simulink model "Task_Stable"  (R2023a)
settings: Solver=VariableStepAuto  StartTime=0.0  StopTime=10.0  RelTol=1e-3
libraries: cstblocks x3
settings Model: Creator=aalia  LastModifiedBy=aalia

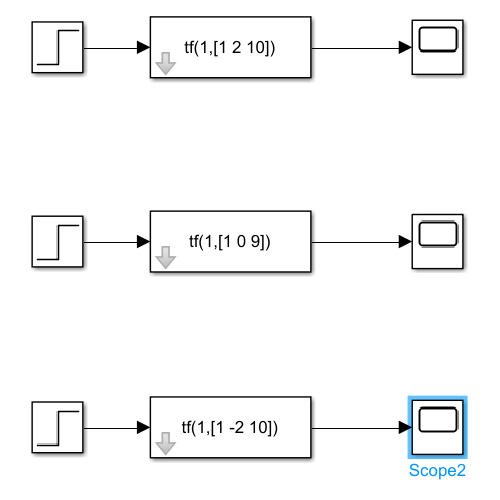
[thumbnail: Simulink's stored preview of the top-level diagram]
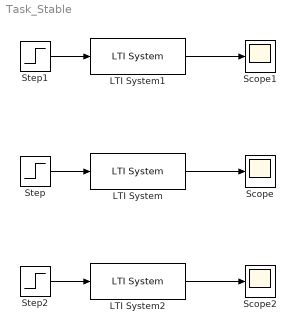
== system Task_Stable ==
  LTI System : cstblocks/LTI System  sys=tf(1,[1 0 9])  IC=[]
  LTI System1 : cstblocks/LTI System  sys=tf(1,[1 2 10])  IC=[]
  LTI System2 : cstblocks/LTI System  sys=tf(1,[1 -2 10])  IC=[]
  Scope : Scope
  Scope1 : Scope
  Scope2 : Scope
  Step : Step  SampleTime=0
  Step1 : Step  SampleTime=0
  Step2 : Step  SampleTime=0
  wires:
  Step/1 -> LTI System/1
  LTI System/1 -> Scope/1
  Step1/1 -> LTI System1/1
  LTI System1/1 -> Scope1/1
  Step2/1 -> LTI System2/1
  LTI System2/1 -> Scope2/1
